simulink model "Chua_TxRx_final_2test"  (R2020a)
settings: Solver=VariableStepAuto  StartTime=0.0  StopTime=500  RelTol=1e-3
libraries: dspsigops x1, dspsrcs4 x1
settings Model: Creator=RaviM  LastModifiedBy=RaviM

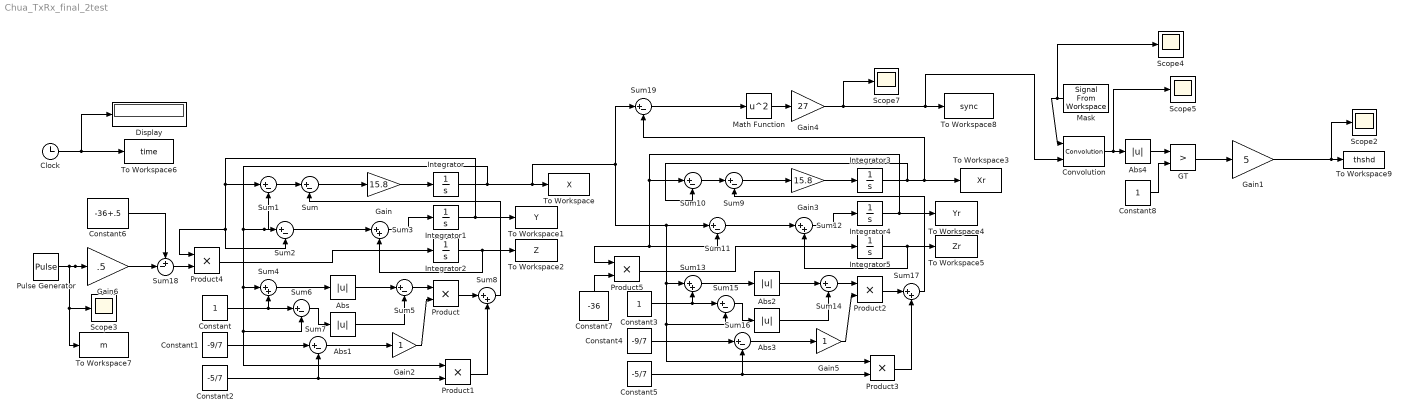
== system Chua_TxRx_final_2test ==
  Abs{,1..4} (5 alike) : Abs
  Clock : Clock
  Constant : Constant
  Constant1 : Constant  Value=-9/7
  Constant2 : Constant  Value=-5/7
  Constant3 : Constant
  Constant4 : Constant  Value=-9/7
  Constant5 : Constant  Value=-5/7
  Constant6 : Constant  Value=-36+.5
  Constant7 : Constant  Value=-36
  Constant8 : Constant
  Convolution : dspsigops/Convolution  domain=Time  roundingMode=Floor  overflowMode=off  outputDataTypeStr=Inherit: Same as accumulator  outputMin=[]  outputMax=[]  outputLastDataTypeStr=Inherit: Same as accumulator
      settings: SourceProductBaseCode=DS
  Display : Display
      settings: Decimation=5
  GT : RelationalOperator  Operator=>  OutDataTypeStr=boolean  RndMeth=Ceiling
  Gain : Gain  Gain=15.8
  Gain1 : Gain  Gain=5
  Gain2 : Gain
  Gain3 : Gain  Gain=15.8
  Gain4 : Gain  Gain=27
  Gain5 : Gain
  Gain6 : Gain  Gain=.5
  Integrator{,1..5} (6 alike) : Integrator  InitialCondition=0.1
  Mask : dspsrcs4/Signal From Workspace  X=mask  Ts=1  nsamps=1  OutputAfterFinalValue=Setting to zero  ignoreOrWarnInputAndFrameLengths=off  OutputFrames=off
  Math Function : Math  Operator=square  SignedPower=on  SaturateOnIntegerOverflow=on
  Product{,1..5} (6 alike) : Product
  Pulse Generator : DiscretePulseGenerator  PulseType=Time based  Amplitude=5  Period=100  PulseWidth=50  PhaseDelay=50
  Scope{2..5,7} (5 alike) : Scope
  Sum{,1..2,5..7,9..11,14..16,19} (13 alike) : Sum  Inputs=|+-
  Sum{3..4,8,12..13,17} (6 alike) : Sum  Inputs=|++
  Sum18 : Sum  Inputs=+-|
  To Workspace : ToWorkspace  VariableName=X  SaveFormat=Timeseries  SampleTime=-1
  To Workspace1 : ToWorkspace  VariableName=Y  SaveFormat=Timeseries  SampleTime=-1
  To Workspace2 : ToWorkspace  VariableName=Z  SaveFormat=Timeseries  SampleTime=-1
  To Workspace3 : ToWorkspace  VariableName=Xr  SaveFormat=Timeseries  SampleTime=-1
  To Workspace4 : ToWorkspace  VariableName=Yr  SaveFormat=Timeseries  SampleTime=-1
  To Workspace5 : ToWorkspace  VariableName=Zr  SaveFormat=Timeseries  SampleTime=-1
  To Workspace6 : ToWorkspace  VariableName=time  SampleTime=-1
  To Workspace7 : ToWorkspace  VariableName=m  SampleTime=-1
  To Workspace8 : ToWorkspace  VariableName=sync  SampleTime=-1
  To Workspace9 : ToWorkspace  VariableName=thshd  SaveFormat=Timeseries  SampleTime=-1
  wires:
  Sum5/1 -> Product/1
  Product4/1 -> Integrator2/1
  Sum3/1 -> Integrator1/1
  Gain2/1 -> Product/2
  Abs1/1 -> Sum5/2
  Sum2/1 -> Sum3/1
  Constant1/1 -> Sum7/1
  Gain/1 -> Integrator/1
  Constant/1 -> Sum6/1, Sum4/2
  Abs/1 -> Sum5/1
  Sum1/1 -> Sum/1
  Product/1 -> Sum8/1
  Product1/1 -> Sum8/2
  Sum6/1 -> Abs1/1
  Sum4/1 -> Abs/1
  Constant2/1 -> Product1/2, Sum7/2
  Sum8/1 -> Sum/2
  Sum7/1 -> Gain2/1
  Integrator2/1 -> Sum3/2, To Workspace2/1
  Sum/1 -> Gain/1
  Sum14/1 -> Product2/1
  Product5/1 -> Integrator5/1
  Sum12/1 -> Integrator4/1
  Gain5/1 -> Product2/2
  Abs3/1 -> Sum14/2
  Sum11/1 -> Sum12/1
  Constant4/1 -> Sum16/1
  Gain3/1 -> Integrator3/1
  Constant3/1 -> Sum15/1, Sum13/2
  Abs2/1 -> Sum14/1
  Sum10/1 -> Sum9/1
  Product2/1 -> Sum17/1
  Product3/1 -> Sum17/2
  Sum15/1 -> Abs3/1
  Sum13/1 -> Abs2/1
  Constant5/1 -> Product3/2, Sum16/2
  Sum17/1 -> Sum9/2
  Sum16/1 -> Gain5/1
  Integrator5/1 -> Sum12/2, To Workspace5/1
  Sum9/1 -> Gain3/1
  Constant6/1 -> Sum18/1
  Sum18/1 -> Product4/2
  Pulse Generator/1 -> Gain6/1, Scope3/1, To Workspace7/1
  Gain6/1 -> Sum18/2
  Clock/1 -> Display/1, To Workspace6/1
  Integrator1/1 -> Sum2/2, Product4/1, Sum1/1, To Workspace1/1
  Integrator4/1 -> Sum11/2, Product5/1, Sum10/1, To Workspace4/1
  Constant7/1 -> Product5/2
  Sum19/1 -> Math Function/1
  Integrator3/1 -> To Workspace3/1, Sum19/2, Sum10/2
  Math Function/1 -> Gain4/1
  Integrator/1 -> Product1/1, Sum6/2, Sum4/1, Sum1/2, Sum2/1, Sum19/1, Sum15/2, Product3/1, Sum13/1, Sum11/1, To Workspace/1
  Gain4/1 -> Scope7/1, Convolution/2, To Workspace8/1
  Mask/1 -> Scope4/1, Convolution/1
  Gain1/1 -> To Workspace9/1, Scope2/1
  Abs4/1 -> GT/1
  GT/1 -> Gain1/1
  Constant8/1 -> GT/2
  Convolution/1 -> Scope5/1, Abs4/1
